simulink model "max31855_task"  (Simulink 3.00)
libraries: mathlib x3, speclib x1, arclib x1

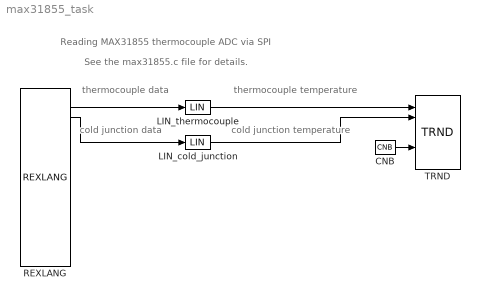
== system max31855_task ==
  note: Reading MAX31855 thermocouple ADC via SPI
  note: See the max31855.c file for details.
  note: thermocouple data
  note: thermocouple temperature
  note: cold junction
      | data
  note: cold junction
      | temperature
  CNB : mathlib/CNB  YCN=on
  LIN_cold_junction : mathlib/LIN  u1=2032  y1=127  u2=-880  y2=-55
  LIN_thermocouple : mathlib/LIN  u1=6400  y1=1600  u2=-1000  y2=-250
  REXLANG : speclib/REXLANG  SystemSampleTime=-1  tab_matlab=BASIC  srcname=max31855.c  srctype=1: STL  stack=0  debug=1: No check  p0=0  p1=0  p2=0  p3=0  p4=0  p5=0  p6=0  p7=0  p8=0  p9=0  p10=0  p11=0  p12=0  p13=0  p14=0  p15=0  fname=/dev/spidev0.0
  TRND : arclib/TRND  n=4  l=1000  btype=8: Double  ptype1=1: Store  ptype2=1: Store  ptype3=1: Store  ptype4=1: Store  pfac=1  afac=0  arc=0  id=1  Title=Measured values
  wires:
  CNB/1 -> TRND/5
  LIN_cold_junction/1 -> TRND/2
  LIN_thermocouple/1 -> TRND/1
  REXLANG/2 -> LIN_thermocouple/1
  REXLANG/3 -> LIN_cold_junction/1
